simulink model "modell2"  (R2021a)
settings: Solver=FixedStepAuto  StartTime=0.0  StopTime=tfinal  FixedStep=tstep  RelTol=1e-3
undefined symbols (not defined in the file): A_Modell, B_Modell, C_Modell, D_Modell, tfinal, ttrans, X0
libraries: simulink x1
settings Model: Creator=62958  LastModifiedBy=62958
settings SolverCC: AlgebraicLoopSolver=TrustRegion
settings DataIOCC: LoggingToFile=on
settings DebuggingCC: SFMachineParentedDataDiag=warning

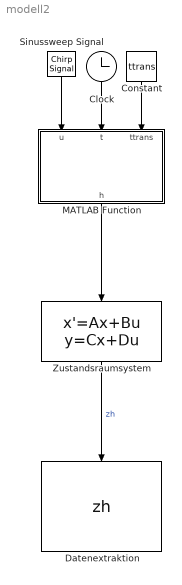
== system modell2 ==
  Clock : Clock
  Constant : Constant  Value=ttrans
  Datenextraktion : ToWorkspace  VariableName=zh  SaveFormat=Timeseries  SampleTime=-1
  MATLAB Function : MATLAB Function  TreatAsAtomicUnit=on
  Sinussweep Signal : simulink/Sources/Chirp Signal  f1=f0  T=tfinal  f2=f1
  Zustandsraumsystem : StateSpace  A=A_Modell  B=B_Modell  C=C_Modell  D=D_Modell  InitialCondition=X0
  wires:
  Sinussweep Signal/1 -> MATLAB Function/1(u)
  Zustandsraumsystem/1 -> Datenextraktion/1  "zh"
  MATLAB Function/1(h) -> Zustandsraumsystem/1
  Clock/1 -> MATLAB Function/2(t)
  Constant/1 -> MATLAB Function/3(ttrans)

== matlab function modell2/MATLAB Function ==
  data: u input; h output; t input; ttrans input
function h = fcn(u,t,ttrans)
if (t<=ttrans)
    h=u;
else
    h=u*ttrans/t;
end
